simulink model "IC80025"  (Simulink 9.0)
settings: Solver=ode23tb  StartTime=0.0  StopTime=0.5  MaxStep=5e-6  RelTol=1e-3  EnableMultiTasking=on
undefined symbols (not defined in the file or in its folder): Ion, Lithium, sigbuilder_block
libraries: powerlib x23, simulink x3, electricdrivelib x1
settings Model: Creator=Administrator  LastModifiedBy=dell
settings SolverCC: AlgebraicLoopSolver=LineSearch
settings DataIOCC: LimitDataPoints=on  SignalLoggingSaveFormat=ModelDataLogs
settings OptimizationCC: ExpressionDepthLimit=2147483647
settings DebuggingCC: SolverPrmCheckMsg=warning  FcnCallInpInsideContextMsg=warning  StateNameClashWarn=warning
settings GRTTargetCC: GeneratePreprocessorConditionals=Disable all  CombineOutputUpdateFcns=off  GRTInterface=on

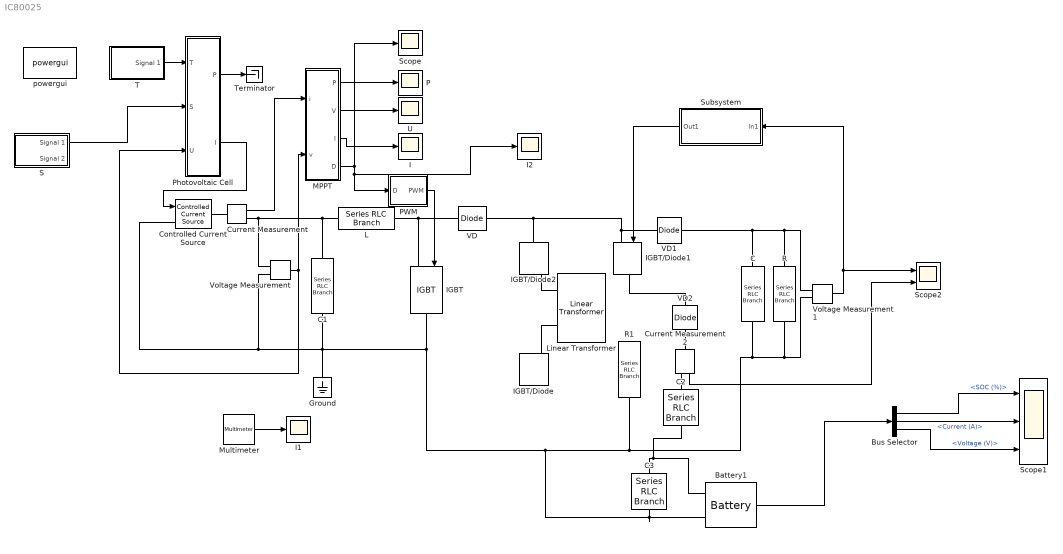
== system IC80025 ==
  Battery1 : electricdrivelib/Extra Sources/Battery  BatType=Lithium-Ion  ShowTempParam=off  ThermalPreset=no  ShowAgeParam=off  NomV=7.2  NomQ=5.4  SOC=80  Batt_Tr=30  PresetModel=off  MaxQ=5.4  MinV=5.4  FullV=8.3807  Dis_rate=2.3478  R=0.013333  Normal_OP=4.8835  expZone="[7.7788      0.2653]"  current=[6.5 13 32.5]  Units=Ampere-hour  Tci=20  NomT=20  T2=-30  MaxQ2=4.8  FullV2=7.1  Normal_OP2=5.655  expZone2="[6.58           1]"  Rca=0.6  ti=2000  Dp=0  Neq0=0  Tsim=1e6  Ta1=25  Qeol=5.4*0.9  Reol=0.013333*1.2  Char_age=[2.3478, 3]  Dis_age=[2.3478, 10]  N1=1500  N2=10500  N3=1000  N4=1400  Ta2=45  N5=950
  Bus Selector : BusSelector  OutputSignals=SOC (%),Current (A),Voltage (V)
  C : powerlib/Elements/Series RLC Branch  LConnTagsString=__new0  RConnTagsString=__new0  BranchType=C  Resistance=0  Inductance=0  SetiL0=off  InitialCurrent=0  Capacitance=300e-5  Setx0=on  InitialVoltage=0  Measurements=None
  C1 : powerlib/Elements/Series RLC Branch  LConnTagsString=__new0  RConnTagsString=__new0  BranchType=C  Resistance=0  Inductance=0  SetiL0=off  InitialCurrent=0  Capacitance=300e-6  Setx0=off  InitialVoltage=0  Measurements=None
  C2 : powerlib/Elements/Series RLC Branch  LConnTagsString=__new0  RConnTagsString=__new0  BranchType=L  Resistance=0  Inductance=1/120  SetiL0=off  InitialCurrent=0  Capacitance=300e-5  Setx0=on  InitialVoltage=0  Measurements=None
  C3 : powerlib/Elements/Series RLC Branch  LConnTagsString=__new0  RConnTagsString=__new0  BranchType=C  Resistance=0  Inductance=0  SetiL0=off  InitialCurrent=0  Capacitance=300e-5  Setx0=on  InitialVoltage=0  Measurements=None
  Controlled Current Source : powerlib/Electrical Sources/Controlled Current Source  Initialize=on  Source_Type=DC  Amplitude=0  Phase=0  Frequency=0  Measurements=None
  Current Measurement : powerlib/Measurements/Current Measurement  PhasorSimulation=off  OutputType=Complex  PSBequivalent=0
  Current Measurement2 : powerlib/Measurements/Current Measurement  PhasorSimulation=off  OutputType=Complex  PSBequivalent=0
  Ground : powerlib/Elements/Ground  LConnTagsString=a
  I : Scope
  I1 : Scope
  I2 : Scope
  IGBT : powerlib/Power Electronics/IGBT  Ron=0.00000001  Lon=0  Vf=1  Tf=1e-6  Tt=2e-6  IC=0  Rs=1e5  Cs=inf  Measurements=off
  IGBT/Diode : powerlib/Power Electronics/IGBT//Diode  Ron=1e-3  Rs=1e5  Cs=inf  Measurements=off
  IGBT/Diode1 : powerlib/Power Electronics/IGBT//Diode  Ron=1e-3  Rs=1e5  Cs=inf  Measurements=off
  IGBT/Diode2 : powerlib/Power Electronics/IGBT//Diode  Ron=1e-3  Rs=1e5  Cs=inf  Measurements=off
  L : powerlib/Elements/Series RLC Branch  LConnTagsString=__new0  RConnTagsString=__new0  BranchType=L  Resistance=0  Inductance=200e-6  SetiL0=off  InitialCurrent=1  Capacitance=inf  Setx0=off  InitialVoltage=0  Measurements=None
  Linear Transformer : powerlib/Elements/Linear Transformer  UNITS=pu  NominalPower=[ 250e6 60 ]  winding1="[ 735e3  0.002  0.08 ]"  winding2="[ 315e3  0.002  0.08 ]"  ThreeWindings=off  winding3=[ 315e3 0.002 0.08 ]  RmLm=[ 500 500 ]  Measurements=None  DataType=off
  MPPT : Subsystem
  Multimeter : powerlib/Measurements/Multimeter  PhasorSimulation=off  OutputType=Complex  sel=1  L=2  Gain=1  yselected={'Ub: R'};  PSBOutputType=1  PSBequivalent=0  AxesSetting=[0,0.1,-100,100]  Display=0  SavedBlockNames=-11
  P : Scope
  PWM : Subsystem
  Photovoltaic Cell : Subsystem  mask(Photovoltaic Cell){a=0.00398, b=0.0821, Rs=0.5, Isc=1, Uoc=21.7, Im=0.91, Um=17.6, Sref=1000, Tref=25}
  R : powerlib/Elements/Series RLC Branch  LConnTagsString=__new0  RConnTagsString=__new0  BranchType=R  Resistance=30  Inductance=100e-6  SetiL0=off  InitialCurrent=0  Capacitance=inf  Setx0=off  InitialVoltage=0  Measurements=Branch voltage
  R1 : powerlib/Elements/Series RLC Branch  LConnTagsString=__new0  RConnTagsString=__new0  BranchType=R  Resistance=0.01  Inductance=100e-6  SetiL0=off  InitialCurrent=0  Capacitance=inf  Setx0=off  InitialVoltage=0  Measurements=Branch voltage
  S : Subsystem  Tag=STV Subsys  LoadFcn=sigbuilder_block('load');  StartFcn=sigbuilder_block('start');  StopFcn=sigbuilder_block('stop');  ClipboardFcn=sigbuilder_block('clipboard');  mask(Sigbuilder block){tuvar=[0:10]}
      mask help: Sigbuilder GUI
      mask init:
      | if ~strcmp(get_param(bdroot(gcbh),'SimulationStatus'),'stopped') tuvar = sigbuilder_block('maskInit'); end
      settings: CopyFcn=sigbuilder_block('copy');  DeleteFcn=sigbuilder_block('delete');  ModelCloseFcn=sigbuilder_block('modelClose');  PreSaveFcn=sigbuilder_block('preSave');  PauseFcn=sigbuilder_block('pause')  ContinueFcn=sigbuilder_block('continue')  NameChangeFcn=sigbuilder_block('namechange');  OpenFcn=sigbuilder_block('open',[203.4 141.6 519 339.6 ]);  CloseFcn=sigbuilder_block('close');
      mask Display: plot(0, 0, 100, 100,[2, 2, 32, 32, 2], [68, 8, 8, 68, 68],[32, 2], [38, 38], [32, 19, 2],[53, 60, 44], [32, 17, 17, 2],[16, 16, 31, 31]);txt = getActiveGroup(gcbh);text(2, 100, txt,'verticalAlignment', 'top');
  Scope : Scope
  Scope1 : Scope  NumInputPorts=3
  Scope2 : Scope  NumInputPorts=2
  Subsystem : Subsystem
  T : Subsystem  Tag=STV Subsys  LoadFcn=sigbuilder_block('load');  StartFcn=sigbuilder_block('start');  StopFcn=sigbuilder_block('stop');  ClipboardFcn=sigbuilder_block('clipboard');  mask(Sigbuilder block){tuvar=[0:10]}
      mask help: Sigbuilder GUI
      mask init:
      | if ~strcmp(get_param(bdroot(gcbh),'SimulationStatus'),'stopped') tuvar = sigbuilder_block('maskInit'); end
      settings: CopyFcn=sigbuilder_block('copy');  DeleteFcn=sigbuilder_block('delete');  ModelCloseFcn=sigbuilder_block('modelClose');  PreSaveFcn=sigbuilder_block('preSave');  PauseFcn=sigbuilder_block('pause')  ContinueFcn=sigbuilder_block('continue')  NameChangeFcn=sigbuilder_block('namechange');  OpenFcn=sigbuilder_block('open',[142.759 39.1034 519.517 399.724 ]);  CloseFcn=sigbuilder_block('close');
      mask Display: plot(0, 0, 100, 100,[2, 2, 32, 32, 2], [68, 8, 8, 68, 68],[32, 2], [38, 38], [32, 19, 2],[53, 60, 44], [32, 17, 17, 2],[16, 16, 31, 31]);txt = getActiveGroup(gcbh);text(2, 100, txt,'verticalAlignment', 'top');
  Terminator : Terminator
  U : Scope
  VD : powerlib/Power Electronics/Diode  Ron=0.00000001  Lon=0  Vf=0.7  IC=0  UseSnubber=off  Rs=500  Cs=250e-9  Measurements=off
  VD1 : powerlib/Power Electronics/Diode  Ron=0.00000001  Lon=0  Vf=0.7  IC=0  UseSnubber=off  Rs=500  Cs=250e-9  Measurements=off
  VD2 : powerlib/Power Electronics/Diode  Ron=0.00000001  Lon=0  Vf=0.7  IC=0  UseSnubber=off  Rs=500  Cs=250e-9  Measurements=off
  Voltage Measurement : powerlib/Measurements/Voltage Measurement  PhasorSimulation=off  OutputType=Complex  PSBequivalent=0
  Voltage Measurement1 : powerlib/Measurements/Voltage Measurement  PhasorSimulation=off  OutputType=Complex  PSBequivalent=0
  powergui : powerlib/powergui  Priority=1  SimulationMode=Discrete  SampleTime=50e-8  frequency=60  Iterations=50  frequencyindice=0  Pbase=100e6  ErrMax=1e-4  UnitsV=kV  UnitsW=MW  buscounter=0  FunctionMessages=off  echomessages=off  EnableUseOfTLC=off  CurrentSourceSwitches=off  DisableSnubberDevices=off  DisableRonSwitches=off  DisableVfSwitches=off  DisplayEquations=off  SolverType=Tustin/Backward Euler (TBE)  Interpol=off  ExternalGateDelay=off  methode=off  Ts=100  x0status=blocks  SPID=off  SwTol=0  HookPort=off  RestoreLinks=warning  ResistiveCurrentMeasurement=off  Frange=[0:2:500]  Ylog=off  Xlog=on  ShowGrid=off  save=off  variable=ZData  structure=0  ZoomFFT=off  StartTime=0.0  cycles=1  DisplayStyle=1  fundamental=60  FreqAxis=off  MaxFrequency=1000  frequencyindicesteady=1  RmsSteady=1  display=off
  wires:
  Photovoltaic Cell/2(I) -> Controlled Current Source/1
  Voltage Measurement/1 -> Photovoltaic Cell/3(U), MPPT/2(v)
  Photovoltaic Cell/1(P) -> Terminator/1
  T/1(Signal 1) -> Photovoltaic Cell/1(T)
  MPPT/4(D) -> I2/1, PWM/1(D), Scope/1
  MPPT/1(P) -> P/1
  MPPT/2(V) -> U/1
  MPPT/3(I) -> I/1
  PWM/1(PWM) -> IGBT/1
  Current Measurement/1 -> MPPT/1(i)
  Multimeter/1 -> I1/1
  Bus Selector/3 -> Scope1/3  "<Voltage (V)>"
  Bus Selector/1 -> Scope1/1  "<SOC (%)>"
  Bus Selector/2 -> Scope1/2  "<Current (A)>"
  Battery1/1 -> Bus Selector/1
  Voltage Measurement1/1 -> Subsystem/1(In1), Scope2/1
  Subsystem/1(Out1) -> IGBT/Diode1/1
  S/1(Signal 1) -> Photovoltaic Cell/2(S)
  Current Measurement2/1 -> Scope2/2
  connections:
  L/RConn1 -- IGBT/LConn1 -- VD/LConn1
  C/LConn1 -- VD1/RConn1 -- Voltage Measurement1/LConn1 -- R/LConn1
  Voltage Measurement/LConn1 -- Current Measurement/RConn1 -- C1/LConn1 -- L/LConn1
  C1/RConn1 -- Controlled Current Source/LConn1 -- Voltage Measurement/LConn2 -- Ground/LConn1 -- Battery1/LConn2 -- C3/RConn1 -- R1/RConn1 -- C/RConn1 -- Voltage Measurement1/LConn2 -- R/RConn1 -- IGBT/RConn1
  Current Measurement/LConn1 -- Controlled Current Source/RConn1
  VD/RConn1 -- IGBT/Diode1/LConn1 -- VD1/LConn1 -- IGBT/Diode2/RConn1
  Linear Transformer/LConn1 -- IGBT/Diode2/LConn1
  IGBT/Diode/LConn1 -- Linear Transformer/LConn2
  VD2/RConn1 -- Current Measurement2/LConn1
  VD2/LConn1 -- IGBT/Diode1/RConn1
  C2/LConn1 -- Current Measurement2/RConn1
  C2/RConn1 -- Battery1/LConn1 -- C3/LConn1

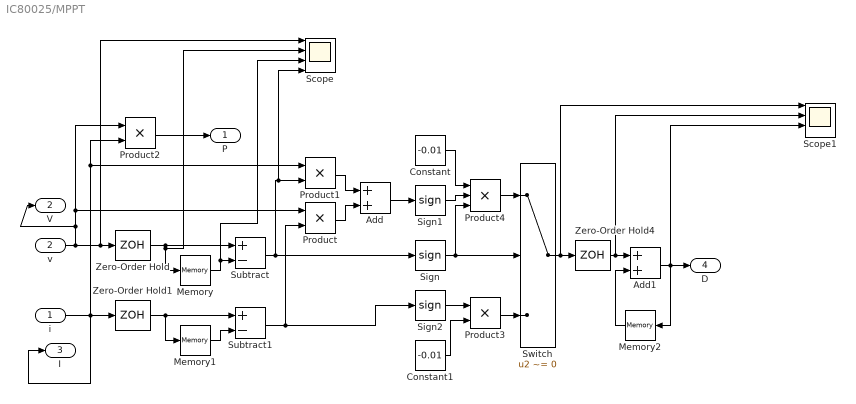
== system IC80025/MPPT ==
  i : Inport
  v : Inport  Port=2
  Add : Sum
  Add1 : Sum
  Constant : Constant  Value=-0.01
  Constant1 : Constant  Value=-0.01
  Memory : Memory
  Memory1 : Memory
  Memory2 : Memory  InitialCondition=1  InheritSampleTime=on
  Product{,1..3} (4 alike) : Product  RndMeth=Zero
  Product4 : Product  Inputs=3  RndMeth=Zero
  Scope : Scope  NumInputPorts=4
  Scope1 : Scope  NumInputPorts=4
  Sign : Signum
  Sign1 : Signum
  Sign2 : Signum
  Subtract : Sum  Inputs=+-
  Subtract1 : Sum  Inputs=+-
  Switch : Switch  Criteria=u2 ~= 0
  Zero-Order Hold : ZeroOrderHold  SampleTime=0.0005
  Zero-Order Hold1 : ZeroOrderHold  SampleTime=0.0005
  Zero-Order Hold4 : ZeroOrderHold  SampleTime=0.0005
  P : Outport
  V : Outport  Port=2
  I : Outport  Port=3
  D : Outport  Port=4
  wires:
  Memory2/1 -> Add1/2
  Add1/1 -> Scope1/3, D/1, Memory2/1
  Product3/1 -> Switch/3
  Sign/1 -> Switch/2, Product4/3
  Constant1/1 -> Product3/2
  Sign2/1 -> Product3/1
  Constant/1 -> Product4/1
  Sign1/1 -> Product4/2
  Product1/1 -> Add/1
  Product/1 -> Add/2
  Subtract1/1 -> Product/2, Sign2/1
  Product2/1 -> P/1
  Memory1/1 -> Subtract1/2
  Zero-Order Hold1/1 -> Memory1/1, Subtract1/1
  i/1 -> Product2/2, Product1/1, I/1, Zero-Order Hold1/1
  Memory/1 -> Scope/3, Subtract/2
  Zero-Order Hold/1 -> Scope/2, Memory/1, Subtract/1
  v/1 -> Product/1, Product2/1, V/1, Scope/1, Zero-Order Hold/1
  Zero-Order Hold4/1 -> Scope1/2, Add1/1
  Add/1 -> Sign1/1
  Product4/1 -> Switch/1
  Switch/1 -> Scope1/1, Zero-Order Hold4/1
  Subtract/1 -> Sign/1, Scope/4, Product1/2

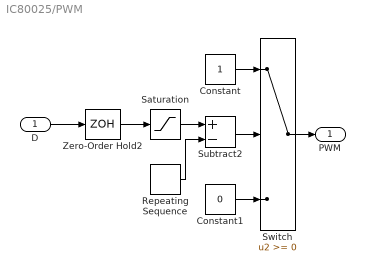
== system IC80025/PWM ==
  D : Inport
  Constant : Constant
  Constant1 : Constant  Value=0
  Repeating Sequence : simulink/Sources/Repeating Sequence  rep_seq_t=[0 0.0001]  rep_seq_y=[0 1]
  Saturation : Saturate  UpperLimit=1  LowerLimit=0
  Subtract2 : Sum  Inputs=+-
  Switch : Switch
  Zero-Order Hold2 : ZeroOrderHold  SampleTime=0.0005
  PWM : Outport
  wires:
  Zero-Order Hold2/1 -> Saturation/1
  Switch/1 -> PWM/1
  Constant1/1 -> Switch/3
  Constant/1 -> Switch/1
  Subtract2/1 -> Switch/2
  Repeating Sequence/1 -> Subtract2/2
  Saturation/1 -> Subtract2/1
  D/1 -> Zero-Order Hold2/1

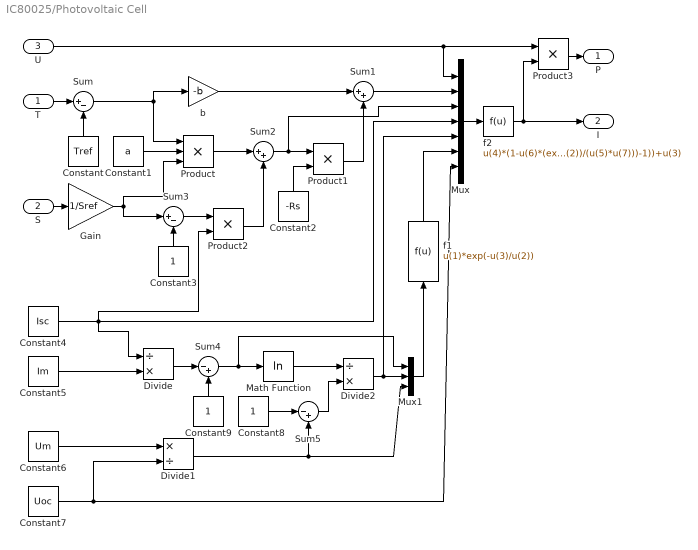
== system IC80025/Photovoltaic Cell ==
  T : Inport
  S : Inport  Port=2
  U : Inport  Port=3
  Constant : Constant  Value=Tref
  Constant1 : Constant  Value=a
  Constant2 : Constant  Value=-Rs
  Constant3 : Constant
  Constant4 : Constant  Value=Isc
  Constant5 : Constant  Value=Im
  Constant6 : Constant  Value=Um
  Constant7 : Constant  Value=Uoc
  Constant8 : Constant
  Constant9 : Constant
  Divide : Product  Inputs=/*
  Divide1 : Product  Inputs=*/
  Divide2 : Product  Inputs=/*
  Gain : Gain  Gain=1/Sref
  Math Function : Math  Operator=log  SaturateOnIntegerOverflow=on
  Mux : Mux  Inputs=7
  Mux1 : Mux  Inputs=3
  Product : Product  Inputs=3  RndMeth=Zero
  Product1 : Product  RndMeth=Zero
  Product2 : Product  RndMeth=Zero
  Product3 : Product  RndMeth=Zero
  Sum : Sum  Inputs=|+-
  Sum1 : Sum  Inputs=|++
  Sum2 : Sum  Inputs=|++
  Sum3 : Sum  Inputs=|+-
  Sum4 : Sum  Inputs=|-+
  Sum5 : Sum  Inputs=|-+
  b : Gain  Gain=-b
  f1 : Fcn  Expr=u(1)*exp(-u(3)/u(2))
  f2 : Fcn  Expr=u(4)*(1-u(6)*(exp((u(1)-u(2))/(u(5)*u(7)))-1))+u(3)
  P : Outport
  I : Outport  Port=2
  wires:
  T/1 -> Sum/1
  Sum/1 -> Product/1, b/1
  b/1 -> Sum1/1
  Constant/1 -> Sum/2
  S/1 -> Gain/1
  Gain/1 -> Product/3, Sum3/1
  Constant1/1 -> Product/2
  Product/1 -> Sum2/1
  Sum2/1 -> Product1/1, Mux/3
  Constant2/1 -> Product1/2
  Sum3/1 -> Product2/1
  Product2/1 -> Sum2/2
  Constant3/1 -> Sum3/2
  Product1/1 -> Sum1/2
  Constant4/1 -> Product2/2, Mux/4, Divide/1
  Sum1/1 -> Mux/2
  U/1 -> Mux/1, Product3/1
  Divide/1 -> Sum4/1
  Constant9/1 -> Sum4/2
  Constant5/1 -> Divide/2
  Constant7/1 -> Divide1/2, Mux/7
  Constant6/1 -> Divide1/1
  Sum4/1 -> Math Function/1, Mux1/1
  Divide1/1 -> Sum5/2, Mux1/3
  Constant8/1 -> Sum5/1
  Sum5/1 -> Divide2/2
  Math Function/1 -> Divide2/1
  Divide2/1 -> Mux1/2, Mux/5
  Mux1/1 -> f1/1
  f1/1 -> Mux/6
  Mux/1 -> f2/1
  Product3/1 -> P/1
  f2/1 -> I/1, Product3/2

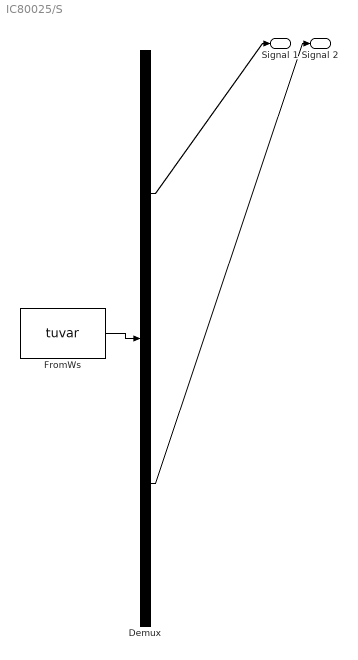
== system IC80025/S ==
  Demux : Demux  Tag=STV Demux  Outputs=2
  FromWs : FromWorkspace  Tag=STV FromWs  VariableName=tuvar  SampleTime=0  SigBuilderData=DataTag0  VnvData=DataTag1
      SigBuilderData=|
      | dataSet.timeRange = [0 0.16]
      | dataSet.name = 'Group 1'
      | sbobj.Groups.Name = 'Group 1'
      | sbobj.Groups.Signals(1).Name = 'Signal 1'
      | sbobj.Groups.Signals(1).XData = [0 0.08 0.08 0.16]
      | sbobj.Groups.Signals(1).YData = [1000 1000 970 970]
      | sbobj.Groups.Signals(2).Name = 'Signal 2'
      | sbobj.Groups.Signals(2).XData = [0 0.0745 0.0745 0.1195 0.1195 0.16]
      | sbobj.Groups.Signals(2).YData = [1000 1000 800 800 600 600]
      | sbobj.Groups.TimeRange = [0 0.16]
  Signal 1 : Outport  Tag=STV Outport
  Signal 2 : Outport  Tag=STV Outport  Port=2
  wires:
  Demux/1 -> Signal 1/1
  FromWs/1 -> Demux/1
  Demux/2 -> Signal 2/1

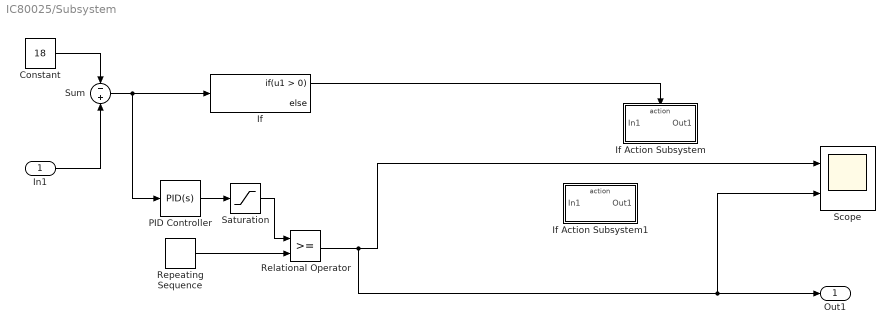
== system IC80025/Subsystem ==
  In1 : Inport
  Constant : Constant  Value=18
  If : If
  If Action Subsystem : Subsystem  TreatAsAtomicUnit=on
  If Action Subsystem1 : Subsystem  TreatAsAtomicUnit=on
  PID Controller : simulink/Continuous/PID Controller  Controller=PID  TimeDomain=Continuous-time  SampleTime=-1  IntegratorMethod=Forward Euler  FilterMethod=Forward Euler  Form=Parallel  UseFilter=on  ControllerParametersSource=internal  P=1  I=1  D=0  N=100  InitialConditionSource=internal  InitialConditionForIntegrator=0  InitialConditionForFilter=0  ExternalReset=none  LimitOutput=off  UpperSaturationLimit=inf  LowerSaturationLimit=-inf  LinearizeAsGain=on  AntiWindupMode=none  Kb=1  TrackingMode=off  Kt=1  PParamMin=[]  PParamMax=[]  IParamMin=[]  IParamMax=[]  DParamMin=[]  DParamMax=[]  NParamMin=[]  NParamMax=[]  KbParamMin=[]  KbParamMax=[]  KtParamMin=[]  KtParamMax=[]  POutMin=[]  POutMax=[]  IOutMin=[]  IOutMax=[]  DOutMin=[]  DOutMax=[]  NOutMin=[]  NOutMax=[]  KbOutMin=[]  KbOutMax=[]  KtOutMin=[]  KtOutMax=[]  IntegratorOutMin=[]  IntegratorOutMax=[]  FilterOutMin=[]  FilterOutMax=[]  SumOutMin=[]  SumOutMax=[]  SumI1OutMin=[]  SumI1OutMax=[]  SumI2OutMin=[]  SumI2OutMax=[]  SumI3OutMin=[]  SumI3OutMax=[]  SumDOutMin=[]  SumDOutMax=[]  SaturationOutMin=[]  SaturationOutMax=[]  IntegratorContinuousStateAttributes=''  IntegratorStateMustResolveToSignalObject=off  IntegratorRTWStateStorageClass=Auto  FilterContinuousStateAttributes=''  FilterStateMustResolveToSignalObject=off  FilterRTWStateStorageClass=Auto  DifferentiatorICPrevScaledInput=0  DifferentiatorOutMin=[]  DifferentiatorOutMax=[]  InitialConditionSetting=State (most efficient)  FilterDiffOutCoefMin=[]  FilterDiffOutCoefMax=[]  SumDenOutMin=[]  SumDenOutMax=[]  SumNumOutMin=[]  SumNumOutMax=[]  ReciprocalOutMin=[]  ReciprocalOutMax=[]  DivideOutMin=[]  DivideOutMax=[]  TunerSelectOption=Transfer Function Based (PID Tuner App)
  Relational Operator : RelationalOperator  OutDataTypeStr=boolean  RndMeth=Simplest
  Repeating Sequence : simulink/Sources/Repeating Sequence  rep_seq_t=[0 0.0001]  rep_seq_y=[0 1]
  Saturation : Saturate  UpperLimit=1  LowerLimit=0
  Scope : Scope  NumInputPorts=2
  Sum : Sum  Inputs=-+
  Out1 : Outport
  wires:
  Constant/1 -> Sum/1
  In1/1 -> Sum/2
  If/1 -> If Action Subsystem/Action
  Sum/1 -> PID Controller/1, If/1
  Repeating Sequence/1 -> Relational Operator/2
  Saturation/1 -> Relational Operator/1
  PID Controller/1 -> Saturation/1
  Relational Operator/1 -> Scope/2, Out1/1, Scope/1

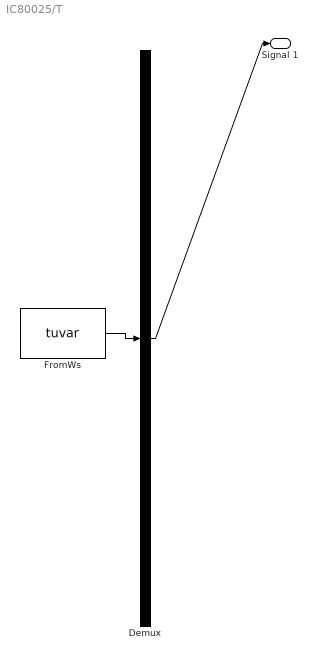
== system IC80025/T ==
  Demux : Demux  Tag=STV Demux  Outputs=1
  FromWs : FromWorkspace  Tag=STV FromWs  VariableName=tuvar  SampleTime=0  SigBuilderData=DataTag2  VnvData=DataTag3
      SigBuilderData=|
      | dataSet.timeRange = [0 0.16]
      | dataSet.name = 'Group 1'
      | sbobj.Groups.Name = 'Group 1'
      | sbobj.Groups.Signals.Name = 'Signal 1'
      | sbobj.Groups.Signals.XData = [0 0.16]
      | sbobj.Groups.Signals.YData = [25 25]
      | sbobj.Groups.TimeRange = [0 0.16]
  Signal 1 : Outport  Tag=STV Outport
  wires:
  FromWs/1 -> Demux/1
  Demux/1 -> Signal 1/1

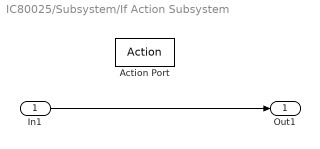
== system IC80025/Subsystem/If Action Subsystem ==
  In1 : Inport
  Action Port : ActionPort  ActionType=then
  Out1 : Outport
  wires:
  In1/1 -> Out1/1

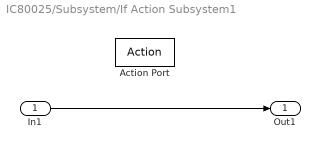
== system IC80025/Subsystem/If Action Subsystem1 ==
  In1 : Inport
  Action Port : ActionPort
  Out1 : Outport
  wires:
  In1/1 -> Out1/1
